simulink model "symulacja"  (R2015a)
settings: Solver=ode45  StartTime=0.0  StopTime=100.0  RelTol=1e-3
undefined symbols (not defined in the file or in its folder): e0, e1, h, K, N, T
libraries: simulink x1
settings Model: Creator=pingwin  LastModifiedBy=pingwin

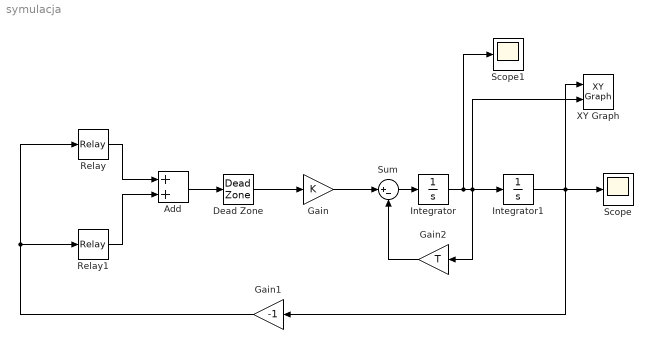
== system symulacja ==
  Add : Sum
  Dead Zone : DeadZone  LowerValue=-N  UpperValue=N  SaturateOnIntegerOverflow=on
  Gain : Gain  Gain=K
  Gain1 : Gain  Gain=-1
  Gain2 : Gain  Gain=T
  Integrator : Integrator  InitialCondition=e1
  Integrator1 : Integrator  InitialCondition=e0
  Relay : Relay  OnSwitchValue=-N  OffSwitchValue=-N-h  OnOutputValue=0  OffOutputValue=-1
  Relay1 : Relay  OnSwitchValue=N+h  OffSwitchValue=N
  Scope : Scope
      settings: SaveName=out_2
  Scope1 : Scope
      settings: SaveName=out_1
  Sum : Sum  Inputs=|+-
  XY Graph : simulink/Sinks/XY Graph  xmin=-10  xmax=10  ymin=-10  ymax=10  st=-1
  wires:
  Relay/1 -> Add/1
  Relay1/1 -> Add/2
  Add/1 -> Dead Zone/1
  Dead Zone/1 -> Gain/1
  Gain1/1 -> Relay/1, Relay1/1
  Gain/1 -> Sum/1
  Gain2/1 -> Sum/2
  Sum/1 -> Integrator/1
  Integrator/1 -> Scope1/1, XY Graph/2, Integrator1/1, Gain2/1
  Integrator1/1 -> Scope/1, Gain1/1, XY Graph/1
